simulink model "Quadcopter_v2"  (R2017b)
settings: Solver=ode23s  StartTime=0.0  StopTime=70  RelTol=1e-3
settings Model: Creator=ANANDA RANGAN N  LastModifiedBy=ANANDA RANGAN N

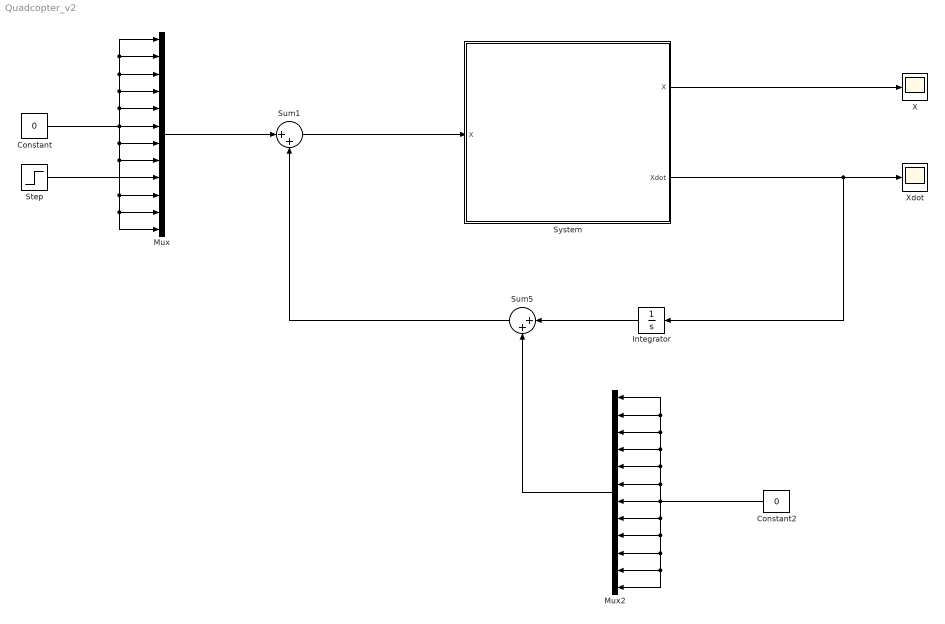
== system Quadcopter_v2 ==
  Constant : Constant  Value=0
  Constant2 : Constant  Value=0
  Integrator : Integrator
  Mux : Mux  Inputs=12
  Mux2 : Mux  Inputs=12
  Step : Step  Time=0.1  Before=0.785398164  After=0  SampleTime=0
  Sum1 : Sum  Inputs=|++
  Sum5 : Sum  Inputs=|++
  System : MATLAB Function  TreatAsAtomicUnit=on
  X : Scope
  Xdot : Scope
  wires:
  Mux/1 -> Sum1/1
  Sum1/1 -> System/1("X ")
  Constant/1 -> Mux/1, Mux/2, Mux/3, Mux/4, Mux/5, Mux/7, Mux/10, Mux/11, Mux/12, Mux/8, Mux/6
  System/1(X) -> X/1
  Constant2/1 -> Mux2/5, Mux2/4, Mux2/3, Mux2/2, Mux2/1, Mux2/6, Mux2/7, Mux2/8, Mux2/9, Mux2/10, Mux2/11, Mux2/12
  Mux2/1 -> Sum5/2
  Integrator/1 -> Sum5/1
  System/2(Xdot) -> Integrator/1, Xdot/1
  Sum5/1 -> Sum1/2
  Step/1 -> Mux/9

== matlab function Quadcopter_v2/System ==
  data: X output; X input; Xdot output
function [X, Xdot] = fcn(X)

%{
  x = ( x, vx, y, vy, z, vy, phi, p, theta, q, psi, r)
  m = mass
  Ix, Iy, Iz = Moment of Inertia along X, Y, Z axes
  Ir = ??
  R = Radius of the wheel
  omega_r
%}
%system parameters
m = 0.468;  
Ix = 0.004856; Iy = 0.004856; Iz = 0.008801;
Ir = 0.00003357; 
omega_r = 50;
R = 0.1025; b = 0.1620;
g = 9.81;

T1 = m*g*sec(X(7))*sec(X(9)); T2 = 0; T3 = 0; T4 = 0; 


%matrix dimension declaration
f = [0;0;0;0;0;0;0;0;0;0;0;0]; 
g1 = [0;0;0;0;0;0;0;0;0;0;0;0]; 
g2 = [0;0;0;0;0;0;0;0;0;0;0;0];
g3 = [0;0;0;0;0;0;0;0;0;0;0;0]; 
g4 = [0;0;0;0;0;0;0;0;0;0;0;0]; 
Xdot = [1;2;3;0;0;0;0;0;0;0;0;0]; 

%variable declaration

x = X(1); y = X(3); z = X(5);
vx = X(2); vy = X(4); vz = X(6);
phi = X(7); p = X(8);
theta = X(9); q = X(10);
psi = X(11); r = X(12);

%intermediate variables
g11 = ((cos(psi)*sin(theta)*cos(phi)) + (sin(psi)*sin(phi)))/m;
g12 = ((sin(psi)*sin(theta)*cos(phi)) - (cos(psi)*sin(phi)))/m;
g13 = cos(theta)*cos(phi)/m;

f(1) = vx;
f(2) = 0;
f(3) = vy;
f(4) = 0;
f(5) = vz;
f(6) = -g;
f(7) = p + (sin(phi)*tan(theta)*q) + (cos(phi)*tan(theta)*r);
f(8) = ((Ir*q*omega_r) + (Iy-Iz)*q*r)/Ix;
f(9) = (cos(phi)*q) - (sin(phi)*r);
f(10) = ((Ir*p*omega_r) + (Iz-Ix)*p*r)/Iy;
f(11) = (sin(phi)*sec(theta)*q) + (cos(phi)*sec(theta)*r);
f(12) = (Ix-Iy)*p*q/Iz;

g1 = [0; g11; 0; g12; 0; g13; 0; 0; 0; 0; 0; 0];
g2 = [0; 0; 0; 0; 0; 0; 0; 1/Ix; 0; 0; 0; 0];
g3 = [0; 0; 0; 0; 0; 0; 0; 0; 0; 1/Iy; 0; 0];
g4 = [0; 0; 0; 0; 0; 0; 0; 0; 0; 0; 0; 1/Iz];

Xdot = f + (g1.*T1) + (g2.*T2) + (g3.*T3) + (g4.*T4);
